simulink model "straightRoadSim3D"  (R2022b)
settings: Solver=VariableStepAuto  StartTime=0.0  StopTime=10.0  RelTol=1e-3
libraries: sim3dautolib x2, sim3dcameralib x1, sim3dlib x1
settings Model: Creator=The MathWorks, Inc.  LastModifiedBy=Administrator
settings SolverCC: AlgebraicLoopSolver=TrustRegion
settings DebuggingCC: UnconnectedInputMsg=warning  UnconnectedOutputMsg=warning  UnconnectedLineMsg=warning  SFMachineParentedDataDiag=warning
settings ModelReferenceCC: EnableRefExpFcnMdlSchedulingChecks=on
settings RTWCC: DLArmComputeVersion=19.05

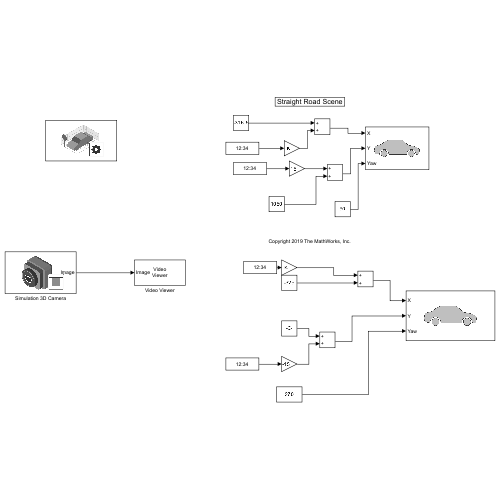
[thumbnail: Simulink's stored preview of the top-level diagram]
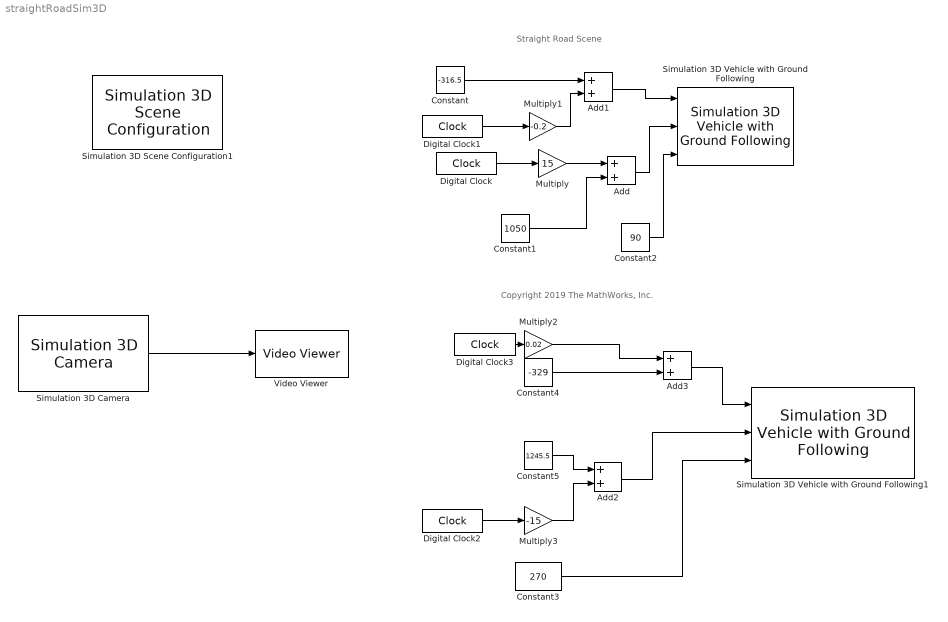
== system straightRoadSim3D ==
  note: Straight Road Scene
  note: Copyright 2019 The MathWorks, Inc.
  Add{,1..3} (4 alike) : Sum
  Constant : Constant  Value=-316.5
  Constant1 : Constant  Value=1050
  Constant2 : Constant  Value=90
  Constant3 : Constant  Value=270
  Constant4 : Constant  Value=-329
  Constant5 : Constant  Value=1245.5
  Digital Clock : DigitalClock  SampleTime=0.01
  Digital Clock1 : DigitalClock  SampleTime=0.01
  Digital Clock2 : DigitalClock  SampleTime=0.02
  Digital Clock3 : DigitalClock  SampleTime=0.02
  Multiply : Gain  Gain=15
  Multiply1 : Gain  Gain=-0.2
  Multiply2 : Gain  Gain=0.02
  Multiply3 : Gain  Gain=-15
  Simulation 3D Camera : sim3dcameralib/Simulation 3D Camera  sensorTag=Sim3dSensor1  sensorId=1  sensorName=Sim3dSensor1  vehTagList={'Scene Origin';'SimulinkVehicle1';'SimulinkVehicle2'}  vehTag=SimulinkVehicle1  mountLoc=Rearview mirror  offsetFlag=off  tmountOffset=[0, 0, 0]  extTmount=off  rmountOffset=[0, 0, 0]  extRmount=off  FocalLength=[320, 320]  OpticalCenter=[640, 480]/2  ImageSize=[480, 640]  RadialDistortion=[0, 0]  TangentialDistortion=[0, 0]  SensorSkew=0  DepthOutportEnabled=off  SemanticOutportEnabled=off  TransformOutportEnabled=off  SampleTime=-1  mountPoint=[0.319999992847443 0 1.19000005722046]  mountOrientation=[0 0 0]  aMode=3  ID=1
  Simulation 3D Scene Configuration1 : sim3dlib/Simulation 3D Scene Configuration  Priority=0  ProjectFormat=Unreal Executable  SceneDesc=Straight road  ProjectName=D:\project\WindowsNoEditor\AutoVrtlEnv.exe  ScenePath=/Game/Maps/HutbCity  UEProjPath=C:\Local\AutoVrtlEnv\AutoVrtlEnv\AutoVrtlEnv.uproject  EnableOpenDRIVE=off  vehTagList={'Scene Origin';'SimulinkVehicle1';'SimulinkVehicle2'}  vehTag=SimulinkVehicle1  OpVisEn=off  Ts=1/60  EnableWindow=on  EnableRemoteAccess=off  EnableWeather=off  SunAltitude=40.0  SunAzimuth=90  clouds=10  wind=1  fog=0  rain=0  EnableGeospatial=off  OriginHeight=200  OriginLatitude=40.744652  OriginLongitude=-73.988864  MapStyle=Aerial  AdditionalAssetIDs=[]  UseAdvancedSunSky=off  SolarTime=11  TimeZone=-5  Day=21  Month=9  Year=2022  UseDaylightSavingTime=on  DSTStartDay=10  DSTStartMonth=3  DSTEndDay=3  DSTEndMonth=11  DSTSwitchHour=2  sensorTag=MainCamera2  sensorId=2  sensorName=MainCamera2  mountLoc=Origin  offsetFlag=off  tmountOffset=[0, 0, 0]  rmountOffset=[0, 0, 0]  HorizontalResolution=1280  VerticalResolution=720  HorizontalFOV=60  mountPoint=[0 0 0]  mountOrientation=[0 0 0]  aMode=3  ID=2  GeoTrigger=Inactive
  Simulation 3D Vehicle with Ground Following : sim3dautolib/Simulation 3D Vehicle with Ground Following  Priority=-1  PassVehMesh=Muscle car  MeshPath=/MathWorksSimulation/Vehicles/Muscle/Meshes/SK_MuscleCar.SK_MuscleCar  TrackWidth=1.9  WheelBase=3  WheelRadius=0.35  VehColor=Red  InitialPos=[-316.5, 1050, 0]  InitialRot=[0, 0, 90]  ActorName=SimulinkVehicle1  SampleTime=-1  ActorType=SimulinkVehicle  ID=1  aMode=3  ActorTag=SimulinkVehicle1  CoordinateScheme=ISO  VehLightsControl=off  HeadlightColor=[ 1, 1, 1 ]  HighBeamIntensity=100000  LowBeamIntensity=60000  HighBeamConeAngle=70  LowBeamConeAngle=70  LeftHeadlightOrientation=[ 0, 0 ]  RightHeadlightOrientation=[ 0, 0 ]  BrakelightIntensity=500  ReverselightIntensity=500  SignallightIntensity=500  SignallightPeriod=1  SignalPulseWidth=50  TransformOutportEnabled=off
  Simulation 3D Vehicle with Ground Following1 : sim3dautolib/Simulation 3D Vehicle with Ground Following  Priority=-1  PassVehMesh=Muscle car  MeshPath=/MathWorksAutomotiveContent/Vehicles/Muscle/Meshes/SK_MuscleCar.SK_MuscleCar  TrackWidth=1.9  WheelBase=3  WheelRadius=0.35  VehColor=Yellow  InitialPos=[-329, 1245.5, 0]  InitialRot=[0, 0, 270]  ActorName=SimulinkVehicle2  SampleTime=-1  ActorType=SimulinkVehicle  ID=2  aMode=3  ActorTag=SimulinkVehicle2  CoordinateScheme=ISO  VehLightsControl=off  HeadlightColor=[ 1, 1, 1 ]  HighBeamIntensity=100000  LowBeamIntensity=60000  HighBeamConeAngle=70  LowBeamConeAngle=70  LeftHeadlightOrientation=[ 0, 0 ]  RightHeadlightOrientation=[ 0, 0 ]  BrakelightIntensity=500  ReverselightIntensity=500  SignallightIntensity=500  SignallightPeriod=1  SignalPulseWidth=50  TransformOutportEnabled=off
      settings: LibrarySourceBlock=drivingsim3d/Simulation 3D Vehicle with Ground Following
  Video Viewer : VideoViewer  FigPos=[61 1240 1920 937]
  wires:
  Constant2/1 -> Simulation 3D Vehicle with Ground Following/3
  Simulation 3D Camera/1 -> Video Viewer/1
  Digital Clock/1 -> Multiply/1
  Multiply/1 -> Add/1
  Constant1/1 -> Add/2
  Add/1 -> Simulation 3D Vehicle with Ground Following/2
  Digital Clock1/1 -> Multiply1/1
  Constant/1 -> Add1/1
  Multiply1/1 -> Add1/2
  Add1/1 -> Simulation 3D Vehicle with Ground Following/1
  Constant3/1 -> Simulation 3D Vehicle with Ground Following1/3
  Digital Clock2/1 -> Multiply3/1
  Constant5/1 -> Add2/1
  Multiply3/1 -> Add2/2
  Add2/1 -> Simulation 3D Vehicle with Ground Following1/2
  Digital Clock3/1 -> Multiply2/1
  Constant4/1 -> Add3/2
  Multiply2/1 -> Add3/1
  Add3/1 -> Simulation 3D Vehicle with Ground Following1/1
